simulink library "sysgenTestbenchLibrary"  (Simulink 6.1)
undefined symbols (not defined in the file or in its folder): magnitude
libraries: dspsigops x4, dspsigattribs x3, dspsrcs4 x2, dspbuff3 x2, dsparch3 x2, dspxfrm3 x2
settings Model: LastModifiedBy=annr

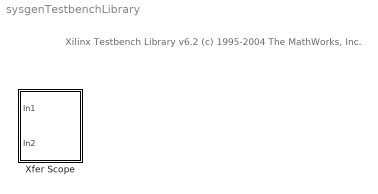
== system sysgenTestbenchLibrary ==
  note: Xilinx Testbench Library v6.2
      | (c) 1995-2004  The MathWorks, Inc.
  Xfer Scope : Subsystem  TreatAsAtomicUnit=on  mask(Xfer Scope){ScopeProperties=off, Domain=Frequency, HorizSpan=1, UseBuffer=on, BufferSize=512, Overlap=64, inpFftLenInherit=off, FFTlength=512, numAvg=500, DisplayProperties=off, AxisGrid=on, Memory=off, FrameNumber=on, AxisLegend=off, AxisZoom=off, OpenScopeAtSimStart=on, OpenScopeImmediately=off, FigPos=[500 200 600 300], AxisProperties=off, XUnits=Hertz, XRange=[0...Fs/2], InheritXIncr=on, XIncr=1, XLabel=Samples, YUnits=dB, YMin=-100, YMax=20, YLabel=Magnitude, dB, LineProperties=on, LineDisables=, LineStyles=, LineMarkers=, LineColors=[0.1 0.2 0.7]|[0.6 0.2 0.1]|[0.1 0.6 0.1]}
      mask prompts: ScopeProperties "_______ Scope properties _______"; Domain "Input domain:"; HorizSpan "Time display span (number of frames):"; UseBuffer "Buffer input"; BufferSize "Buffer size:"; Overlap "Buffer overlap:"; inpFftLenInherit "Specify FFT length"; FFTlength "FFT length:"; numAvg "Number of spectral averages:"; DisplayProperties "_______ Display properties _______"; AxisGrid "Show grid"; Memory "Persistence"; FrameNumber "Frame number"; AxisLegend "Channel legend"; AxisZoom "Compact display"; OpenScopeAtSimStart "Open scope at start of simulation"; OpenScopeImmediately "Open scope immediately"; FigPos "Scope position:"; AxisProperties "_______ Axis properties _______"; XUnits "Frequency units:"; XRange "Frequency range:"; InheritXIncr "Inherit sample increment from input"; XIncr "Sample time of original time series:"; XLabel "X-axis title:"; YUnits "Amplitude scaling:"; YMin "Minimum Y-limit:"; YMax "Maximum Y-limit:"; YLabel "Y-axis title:"; LineProperties "_______ Line properties _______"; LineDisables "Line visibility:"; LineStyles "Line styles:"; LineMarkers "Line markers:"; LineColors "Line colors:"
      mask help:
      | Computes a non-biased transfer function estimation by using
      | the ratio of the cross spectrum between the excitation and response
      | channels, and the autospectrum of the excitation channel.
      |
      | X= channel 1 = DUT excitation (discrete time random noise is best)
      | Y= channel 2 = DUT response from DUT
      |
      | Displays xfer function magnitude in linear or dB format.
      mask init:
      | [x,y,str] = xferscope1('icon');
      | s = xferscope1('init');
      settings: CopyFcn=sdspfscope2([],[],[],'BlockCopy');  DeleteFcn=sdspfscope2([],[],[],'BlockDelete');  NameChangeFcn=sdspfscope2([],[],[],'NameChange');  RTWSystemCode=Function
      mask Help:
      | Use a broad band discrete time excitation and apply it to both
      | analyzer the upper input port and the (discrete time) Device Under Test input.
      | Connect the discrete time DUT response to the lower input port.
      | Averaging of circa 100 produces good results.
      | 
      | The measurement results will be unbiased as long as the excitation
      | does not have noise which is correlated with noise in the response channel.
      | 
      | 
      | RAB 01/28/02
      mask StyleString: checkbox,popup(Time|Frequency|User-defined),edit,checkbox,edit,edit,checkbox,edit,edit,checkbox,checkbox,checkbox,checkbox,checkbox,checkbox,checkbox,checkbox,edit,checkbox,popup(Hertz|rad/sec),popup([0...Fs/2]|[-Fs/2...Fs/2]|[0...Fs]),checkbox,edit,edit,popup(Magnitude|dB),edit,edit,edit,checkbox,edit,edit,edit,edit
      mask CallbackString: dspblkbfftscope2('dynamic','ScopeProperties')|||dspblkbfftscope2('dynamic','useBuffer');|||dspblkbfftscope2('dynamic','FftLenCheckbox');|||dspblkbfftscope2('dynamic','DisplayProperties');|||||||dspblkbfftscope2('dynamic','OpenScope');||dspblkbfftscope2('dynamic','AxisProperties');|||dspblkbfftscope2('dynamic','InheritXIncr');|||||||dspblkbfftscope2('dynamic','LineProperties');||||
      mask Display: plot(x,y); text(14,20,str);

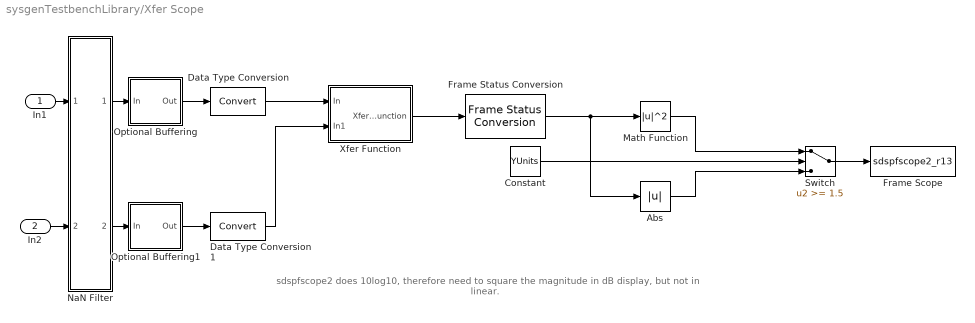
== system sysgenTestbenchLibrary/Xfer Scope ==
  note: sdspfscope2 does 10log10, therefore need to square the magnitude in dB
      | display, but not in linear.
  In1 : Inport  Port=1  LatchInput=off
  In2 : Inport  Port=2  LatchInput=off
  Abs : Abs  SaturateOnIntegerOverflow=on
  Constant : Constant  Value=YUnits
  Data Type Conversion : DataTypeConversion  OutDataTypeMode=double  SaturateOnIntegerOverflow=on  RndMeth=Zero
  Data Type Conversion1 : DataTypeConversion  OutDataTypeMode=double  SaturateOnIntegerOverflow=on  RndMeth=Zero
  Frame Scope : S-Function  FunctionName=sdspfscope2_r13  Parameters=s
  Frame Status Conversion : dspsigattribs/Frame Status Conversion  growRefPort=off  outframe=Sample-based
  Math Function : Math  Operator=magnitude^2  SaturateOnIntegerOverflow=on
  NaN Filter : Subsystem
  Optional Buffering : Subsystem  mask(Replaceable Contents){oname=Buffer, osrc=dspbuff3/Buffer, oargs={'N','BufferSize','V','Overlap','ic','0'}, replace=strcmp(UseBuffer,'off')}
      mask prompts: oname "Relative name of blocks to replace:"; osrc "Simulink path to each source block:"; oargs "Parameter/value pairs to each block:"; replace "Replace with short-circuit:"
      mask help: Configurable subsystem holding blocks which may be replaced by virtual short-circuits (muxes) when not needed.
      mask init:
      | opts.name = oname; opts.src = osrc; opts.args = oargs;
      | dspskipblk(gcb,opts,replace);
  Optional Buffering1 : Subsystem  mask(Replaceable Contents){oname=Buffer, osrc=dspbuff3/Buffer, oargs={'N','BufferSize','V','Overlap','ic','0'}, replace=strcmp(UseBuffer,'off')}
      mask prompts: oname "Relative name of blocks to replace:"; osrc "Simulink path to each source block:"; oargs "Parameter/value pairs to each block:"; replace "Replace with short-circuit:"
      mask help: Configurable subsystem holding blocks which may be replaced by virtual short-circuits (muxes) when not needed.
      mask init:
      | opts.name = oname; opts.src = osrc; opts.args = oargs;
      | dspskipblk(gcb,opts,replace);
  Switch : Switch  Threshold=1.5  SaturateOnIntegerOverflow=on  InputSameDT=on
  Xfer Function : Subsystem  mask(Xfer Function){wintype=Hann, Rs=50, beta=5, winsamp=Periodic, inheritFFT=on, fftsize=FFTlength, navg=numAvg}
      mask prompts: wintype "Window type:"; Rs "Stopband attenuation in dB:"; winsamp "Window sampling:"; inheritFFT "Inherit FFT length from input dimensions"; fftsize "FFT length:"; navg "Number of spectral averages:"
      mask init:
      | [x,y,xe]=xfer_function1('icon');
      | xfer_function1('init');
      mask StyleString: popup(Bartlett|Blackman|Boxcar|Chebyshev|Hamming|Hann|Hanning|Kaiser|Triang),edit,edit,popup(Symmetric|Periodic),checkbox,edit,edit
      mask CallbackString: dspblkshorttimefft2||||dspblkshorttimefft2||
      mask Display: text(-3,1.15,'Xfer_Function'); plot((-xe),0,xe,1.3,x,y)
  wires:
  Data Type Conversion/1 -> Xfer Function/1(In)
  Optional Buffering/1(Out) -> Data Type Conversion/1
  Xfer Function/1(Xfer_Function) -> Frame Status Conversion/1
  Frame Status Conversion/1 -> Math Function/1, Abs/1
  Optional Buffering1/1(Out) -> Data Type Conversion1/1
  Data Type Conversion1/1 -> Xfer Function/2(In1)
  Math Function/1 -> Switch/1
  Switch/1 -> Frame Scope/1
  Abs/1 -> Switch/3
  Constant/1 -> Switch/2
  NaN Filter/1(Out1) -> Optional Buffering/1(In)
  NaN Filter/2(Out2) -> Optional Buffering1/1(In)
  In2/1 -> NaN Filter/2(In2)
  In1/1 -> NaN Filter/1(In1)

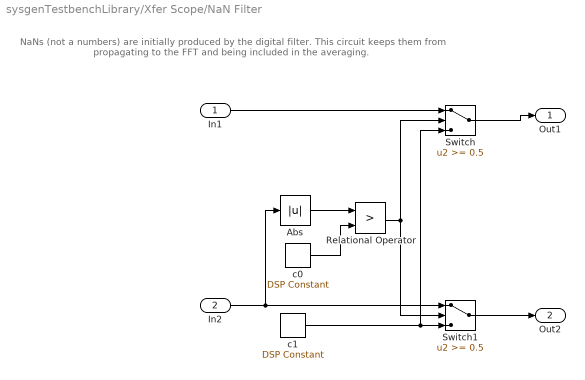
== system sysgenTestbenchLibrary/Xfer Scope/NaN Filter ==
  note: NaNs  (not a numbers) are initially produced by the digital filter.
      | This circuit keeps them from propagating to the FFT and being
      | included in the averaging.
  In1 : Inport  Port=1  LatchInput=off
  In2 : Inport  Port=2  LatchInput=off
  Abs : Abs  SaturateOnIntegerOverflow=on
  Relational Operator : RelationalOperator  Operator=>  InputSameDT=on
  Switch : Switch  Threshold=0.5  SaturateOnIntegerOverflow=on  InputSameDT=on
  Switch1 : Switch  Threshold=0.5  SaturateOnIntegerOverflow=on  InputSameDT=on
  c0 : dspsrcs4/DSP Constant  Value=-inf  SampleMode=Continuous  discreteOutput=Sample-based  continuousOutput=Sample-based  sampTime=1  framePeriod=1  dataType=Inherit from 'Constant value'  wordLen=16  udDataType=sfix(16)  fracBitsMode=Best precision  numFracBits=15  InterpretAs1D=off  Ts=1  FramebasedOutput=off
  c1 : dspsrcs4/DSP Constant  Value=0  SampleMode=Continuous  discreteOutput=Sample-based  continuousOutput=Sample-based  sampTime=1  framePeriod=1  dataType=Inherit from 'Constant value'  wordLen=16  udDataType=sfix(16)  fracBitsMode=Best precision  numFracBits=15  InterpretAs1D=off  Ts=1  FramebasedOutput=off
  Out1 : Outport
  Out2 : Outport  Port=2
  wires:
  In2/1 -> Switch1/1, Abs/1
  In1/1 -> Switch/1
  Switch/1 -> Out1/1
  Switch1/1 -> Out2/1
  Abs/1 -> Relational Operator/1
  c0/1 -> Relational Operator/2
  Relational Operator/1 -> Switch/2, Switch1/2
  c1/1 -> Switch1/3, Switch/3

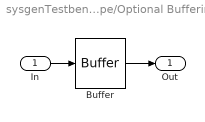
== system sysgenTestbenchLibrary/Xfer Scope/Optional Buffering ==
  In : Inport  Port=1  LatchInput=off
  Buffer : dspbuff3/Buffer  N=BufferSize  V=Overlap  ic=0
  Out : Outport  InitialOutput=0
  wires:
  In/1 -> Buffer/1
  Buffer/1 -> Out/1

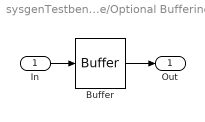
== system sysgenTestbenchLibrary/Xfer Scope/Optional Buffering1 ==
  In : Inport  Port=1  LatchInput=off
  Buffer : dspbuff3/Buffer  N=BufferSize  V=Overlap  ic=0
  Out : Outport  InitialOutput=0
  wires:
  Buffer/1 -> Out/1
  In/1 -> Buffer/1

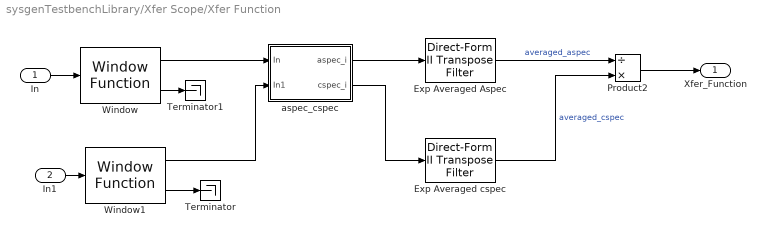
== system sysgenTestbenchLibrary/Xfer Scope/Xfer Function ==
  In : Inport  Port=1  LatchInput=off
  In1 : Inport  Port=2  LatchInput=off
  "Exp Averaged Aspec " : dsparch3/Direct-Form II Transpose Filter  num=-1  den=[abs(navg) (-abs(navg)-1)]  ic=eps
  Exp Averaged cspec : dsparch3/Direct-Form II Transpose Filter  num=-1  den=[abs(navg) (-abs(navg)-1)]  ic=eps
  Product2 : Product  Inputs=/*  SaturateOnIntegerOverflow=on  InputSameDT=on
  Terminator : Terminator
  Terminator1 : Terminator
  Window : dspsigops/Window Function  winmode=Generate and apply window  wintype=Hann  N=64  Rs=Rs  beta=beta  winsamp=Periodic  UserWindow=hamming  OptParams=off  UserParams={1.0}  datatype=Double
  Window1 : dspsigops/Window Function  winmode=Generate and apply window  wintype=Hann  N=64  Rs=Rs  beta=beta  winsamp=Symmetric  UserWindow=hamming  OptParams=off  UserParams={1.0}  datatype=Double
  aspec_cspec : Subsystem  mask(aspec_aspec){fftLenInherit=on, fftsize=fftsize}
      mask prompts: fftLenInherit "Inherit FFT length from input dimensions"; fftsize "FFT length:"
      mask init:
      | aspec_cspec1('init');aspec_cspec1('update'); str='aspec_cspec';
      mask CallbackString: dspblkmagfft2;|
      mask Display: disp(str);
  Xfer_Function : Outport  InitialOutput=0
  wires:
  "Exp Averaged Aspec "/1 -> Product2/1  "averaged_aspec"
  Product2/1 -> Xfer_Function/1
  Window/1 -> aspec_cspec/1(In)
  aspec_cspec/1(aspec_i) -> "Exp Averaged Aspec "/1
  In/1 -> Window/1
  In1/1 -> Window1/1
  Window1/1 -> aspec_cspec/2(In1)
  Window1/2 -> Terminator/1
  aspec_cspec/2(cspec_i) -> Exp Averaged cspec/1
  Window/2 -> Terminator1/1
  Exp Averaged cspec/1 -> Product2/2  "averaged_cspec"

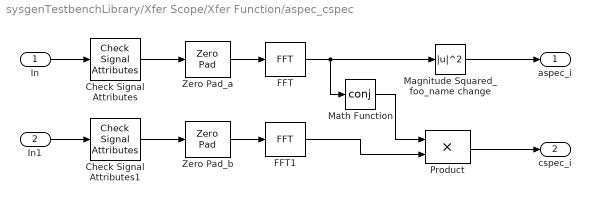
== system sysgenTestbenchLibrary/Xfer Scope/Xfer Function/aspec_cspec ==
  In : Inport  Port=1  LatchInput=off
  In1 : Inport  Port=2  LatchInput=off
  Check Signal Attributes : dspsigattribs/Check Signal Attributes  SigAttribCheckMethod=Matches attributes exactly  Complexity=Ignore  Frame=Sample-based  DimsCheckMethod=Is...  Dimensions=Row vector (2-D)  DatatypeCheckMethod=Ignore  DatatypeGeneral=Boolean  DtypeFloatSpecific=Any floating-point  DtypeFixedSpecific=Any fixed-point  DtypeIntSpecific=Any integer  SampleMode=Ignore
  Check Signal Attributes1 : dspsigattribs/Check Signal Attributes  SigAttribCheckMethod=Matches attributes exactly  Complexity=Ignore  Frame=Sample-based  DimsCheckMethod=Is...  Dimensions=Row vector (2-D)  DatatypeCheckMethod=Ignore  DatatypeGeneral=Boolean  DtypeFloatSpecific=Any floating-point  DtypeFixedSpecific=Any fixed-point  DtypeIntSpecific=Any integer  SampleMode=Ignore
  FFT : dspxfrm3/FFT  CompMethod=Table lookup  TableOpt=Speed  BitRevOrder=off
  FFT1 : dspxfrm3/FFT  CompMethod=Table lookup  TableOpt=Speed  BitRevOrder=off
  Magnitude Squared_foo_name change : Math  Operator=magnitude^2  SaturateOnIntegerOverflow=on
  Math Function : Math  Operator=conj  SaturateOnIntegerOverflow=on
  Product : Product  SaturateOnIntegerOverflow=on  InputSameDT=on
  Zero Pad_a : dspsigops/Zero Pad  padSigAt=End  zpadAlong=None  padNumOutRowsSpecMethod=User-specified  numOutRows=fftsize  padNumOutColsSpecMethod=User-specified  numOutCols=1  trunc_flag=None
  Zero Pad_b : dspsigops/Zero Pad  padSigAt=End  zpadAlong=None  padNumOutRowsSpecMethod=User-specified  numOutRows=fftsize  padNumOutColsSpecMethod=User-specified  numOutCols=1  trunc_flag=None
  aspec_i : Outport
  cspec_i : Outport  Port=2
  wires:
  Check Signal Attributes/1 -> Zero Pad_a/1
  Zero Pad_a/1 -> FFT/1
  FFT/1 -> Math Function/1, Magnitude Squared_foo_name change/1
  In/1 -> Check Signal Attributes/1
  Magnitude Squared_foo_name change/1 -> aspec_i/1
  In1/1 -> Check Signal Attributes1/1
  Check Signal Attributes1/1 -> Zero Pad_b/1
  Zero Pad_b/1 -> FFT1/1
  Math Function/1 -> Product/1
  FFT1/1 -> Product/2
  Product/1 -> cspec_i/1
